simulink model "laplace_sim"  (R2024b)
settings: Solver=VariableStepAuto  StartTime=0.0  StopTime=10  RelTol=1e-3
settings Model: PacingRate=0.500000  Creator=juliawilkosz  LastModifiedBy=juliawilkosz

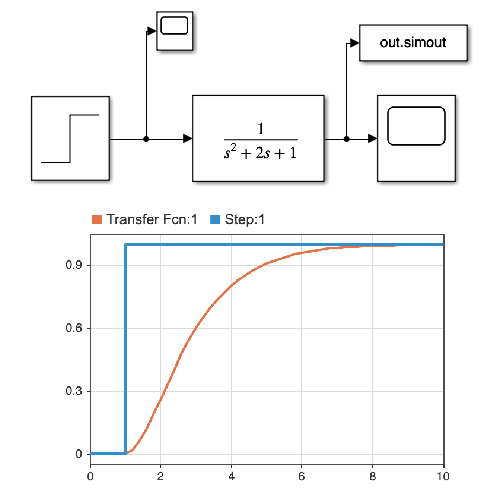
[thumbnail: Simulink's stored preview of the top-level diagram]
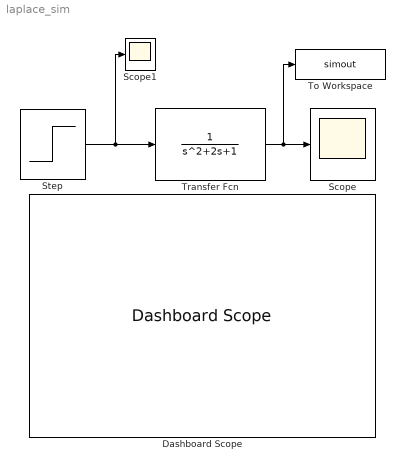
== system laplace_sim ==
  Dashboard Scope : DashboardScope
  Scope : Scope
  Scope1 : Scope
  Step : Step  SampleTime=0
  To Workspace : ToWorkspace  VariableName=simout  SaveFormat=Timeseries  SampleTime=-1
  Transfer Fcn : TransferFcn
  wires:
  Step/1 -> Scope1/1, Transfer Fcn/1
  Transfer Fcn/1 -> To Workspace/1, Scope/1
